simulink model "three_phase_bidirectional_EV_charger_simscape"  (R2019a)
settings: Solver=ode23tb  StartTime=0.0  StopTime=0.2  MaxStep=1e-5  RelTol=1e-5
values from neighbouring files (symbols this model uses):
  C = 33e-6    (= 3.3e-05)    [parameters_for_g2v_closed_loop.m]    (also in parameters_for_v2g_closed_loop.m = 0.002)
  Cf = 300e-3    (= 0.3)    [parameters_for_g2v_closed_loop.m]    (also in parameters_for_v2g_closed_loop.m)
  Co = 2e-3    (= 0.002)    [parameters_for_g2v_closed_loop.m]    (also in parameters_for_v2g_closed_loop.m)
  fline = 50    [parameters_for_g2v_closed_loop.m]    (also in parameters_for_v2g_closed_loop.m)
  fsw_dc = 100e3    (= 100000)    [parameters_for_g2v_closed_loop.m]    (also in parameters_for_v2g_closed_loop.m)
  H = 0.0075    [parameters_for_g2v_closed_loop.m]    (also in parameters_for_v2g_closed_loop.m)
  I = V/R    (= 10)    [parameters_for_g2v_closed_loop.m]    (also in parameters_for_v2g_closed_loop.m = V/(R*(1-D)))
  indicator = 1    [parameters_for_g2v_closed_loop.m]    (also in parameters_for_v2g_closed_loop.m = 0)
  Iqe_max = -Idc_max/K    (= -16.4102564103)    [parameters_for_g2v_closed_loop.m]    (also in parameters_for_v2g_closed_loop.m)
  Kic = Kpc/Tc    (= 4545.45454545)    [parameters_for_g2v_closed_loop.m]    (also in parameters_for_v2g_closed_loop.m)
  Kic_dc = 6749.8    [parameters_for_g2v_closed_loop.m]    (also in parameters_for_v2g_closed_loop.m = 9270.6)
  Kipll = Kpll/Tpll    [parameters_for_g2v_closed_loop.m]    (also in parameters_for_v2g_closed_loop.m)
  Kiv = Kpv/Tv_ac    [parameters_for_g2v_closed_loop.m]    (also in parameters_for_v2g_closed_loop.m)
  Kiv_dc = 15687    [parameters_for_g2v_closed_loop.m]    (also in parameters_for_v2g_closed_loop.m = 1260000)
  Kpc = Kc    (= 32.7272727273)    [parameters_for_g2v_closed_loop.m]    (also in parameters_for_v2g_closed_loop.m)
  Kpc_dc = 0.3    [parameters_for_g2v_closed_loop.m]    (also in parameters_for_v2g_closed_loop.m = 0.29)
  Kpll = (1/Vm)*(1/(alfa_pll*Tsamp_ac))    [parameters_for_g2v_closed_loop.m]    (also in parameters_for_v2g_closed_loop.m)
  Kpv = Kv    [parameters_for_g2v_closed_loop.m]    (also in parameters_for_v2g_closed_loop.m)
  Kpv_dc = 6.9    [parameters_for_g2v_closed_loop.m]    (also in parameters_for_v2g_closed_loop.m = 625.3)
  L = 250e-6    (= 0.00025)    [parameters_for_g2v_closed_loop.m]    (also in parameters_for_v2g_closed_loop.m)
  Lg = 1e-3    (= 0.001)    [parameters_for_g2v_closed_loop.m]    (also in parameters_for_v2g_closed_loop.m)
  Li = 1.6e-3    (= 0.0016)    [parameters_for_g2v_closed_loop.m]    (also in parameters_for_v2g_closed_loop.m)
  Ls = 1e-3    (= 0.001)    [parameters_for_g2v_closed_loop.m]    (also in parameters_for_v2g_closed_loop.m)
  R = V/Iload    (= 50)    [parameters_for_g2v_closed_loop.m]    (also in parameters_for_v2g_closed_loop.m = 1000000)
  Resr = 6e-3    (= 0.006)    [parameters_for_g2v_closed_loop.m]    (also in parameters_for_v2g_closed_loop.m = 0)
  Rf = 0.25    [parameters_for_g2v_closed_loop.m]    (also in parameters_for_v2g_closed_loop.m)
  RL = 10e-3    (= 0.01)    [parameters_for_g2v_closed_loop.m]    (also in parameters_for_v2g_closed_loop.m)
  Rs = 0.5    [parameters_for_g2v_closed_loop.m]    (also in parameters_for_v2g_closed_loop.m)
  T1 = Tsamp_ac/10    (= 5e-06)    [parameters_for_g2v_closed_loop.m]    (also in parameters_for_v2g_closed_loop.m)
  T2 = Tsamp_ac/10    (= 5e-06)    [parameters_for_g2v_closed_loop.m]    (also in parameters_for_v2g_closed_loop.m)
  Tsamp_ac = Tsw_ac/2    (= 5e-05)    [parameters_for_g2v_closed_loop.m]    (also in parameters_for_v2g_closed_loop.m)
  Tsamp_dc = Tsw_dc/2    (= 5e-06)    [parameters_for_g2v_closed_loop.m]    (also in parameters_for_v2g_closed_loop.m)
  V = 500    [parameters_for_g2v_closed_loop.m]    (also in parameters_for_v2g_closed_loop.m = 800)
  Vdc = 800    [parameters_for_g2v_closed_loop.m]    (also in parameters_for_v2g_closed_loop.m)
  Vm = 325    [parameters_for_g2v_closed_loop.m]    (also in parameters_for_v2g_closed_loop.m)
  VM = 4    [parameters_for_g2v_closed_loop.m]    (also in parameters_for_v2g_closed_loop.m)
undefined symbols (not defined in the file or in its folder): Ion, Lithium
libraries: powerlib x58, simulink x9, powerlib_meascontrol x1, electricdrivelib x1
(part 2 of 2)

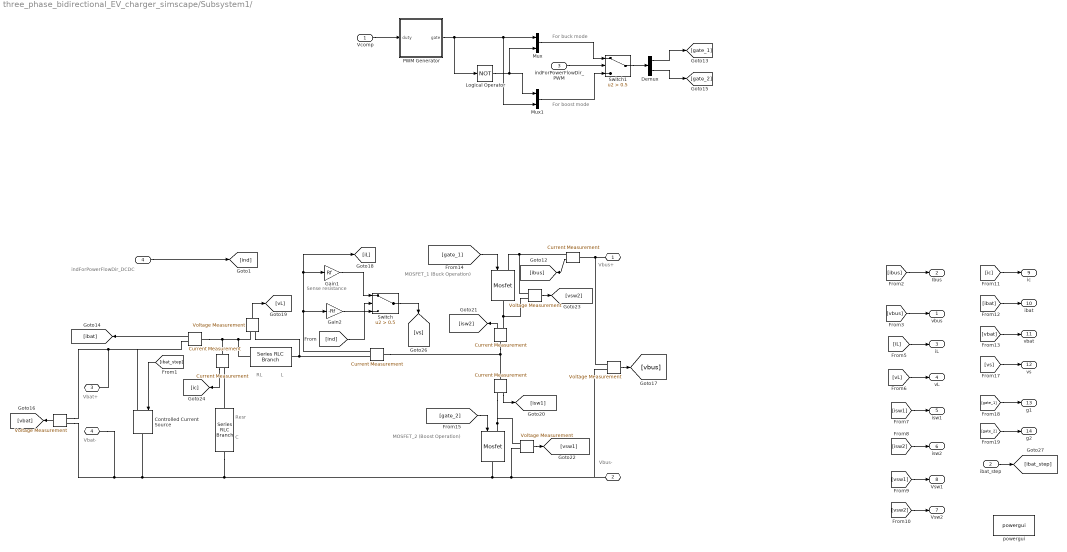
== system three_phase_bidirectional_EV_charger_simscape/Subsystem1/    ==
  note: For buck mode
  note: MOSFET_1
      | (Buck Operation)
  note: MOSFET_2
      | (Boost Operation)
  note: C
  note: Resr
  note: RL
  note: L
  note: Vbat+
  note: Vbat-
  note: Vbus+
  note: Vbus-
  note: For boost mode
  note: indForPowerFlowDir_DCDC
  note: Sense
      | resistance
  Vcomp : Inport
  ibat_step : Inport  Port=2
  indForPowerFlowDir_PWM : Inport  Port=3
  " " : Inport  Port=4
  " " : powerlib/Power Electronics/Mosfet  Ron=Rdson  Lon=0  Rd=0  Vfd=Vf  IC=0  Rs=1e5  Cs=inf  Measurements=off
      settings: SourceProductName=Simscape Electrical
   {,,,} (4 alike) : powerlib/Measurements/Voltage Measurement  PhasorSimulation=off  OutputType=Complex  PSBequivalent=0
      settings: SourceProductName=Simscape Electrical
   {,,,} (4 alike) : powerlib/Measurements/Current Measurement  PhasorSimulation=off  OutputType=Complex  PSBequivalent=0
      settings: SourceProductName=Simscape Electrical
  "    " : powerlib/Elements/Series RLC Branch  LConnTagsString=__new0  RConnTagsString=__new0  BranchType=RC  Resistance=Resr  Inductance=1e-3  SetiL0=off  InitialCurrent=0  Capacitance=C  Setx0=off  InitialVoltage=0  Measurements=None
      settings: SourceProductName=Simscape Electrical
  "        " : powerlib/Measurements/Current Measurement  PhasorSimulation=off  OutputType=Complex  PSBequivalent=0
      settings: SourceProductName=Simscape Electrical
  "          " : powerlib/Power Electronics/Mosfet  Ron=Rdson  Lon=0  Rd=0  Vfd=Vf  IC=0  Rs=1e5  Cs=inf  Measurements=off
      settings: SourceProductName=Simscape Electrical
  " " : powerlib/Elements/Series RLC Branch  LConnTagsString=__new0  RConnTagsString=__new0  BranchType=RL  Resistance=RL  Inductance=L  SetiL0=off  InitialCurrent=0  Capacitance=1e-6  Setx0=off  InitialVoltage=0  Measurements=None
      settings: SourceProductName=Simscape Electrical
  "                                                                                 " : powerlib/Measurements/Current Measurement  PhasorSimulation=off  OutputType=Complex  PSBequivalent=0
      settings: SourceProductName=Simscape Electrical
  "                                                                                                                                        " : powerlib/Measurements/Voltage Measurement  PhasorSimulation=off  OutputType=Complex  PSBequivalent=0
      settings: SourceProductName=Simscape Electrical
  Controlled Current Source : powerlib/Electrical Sources/Controlled Current Source  Initialize=off  Source_Type=AC  Amplitude=0  Phase=0  Frequency=0  Measurements=None
      settings: SourceProductName=Simscape Electrical
  Demux : Demux  Outputs=2
  Gain1 : Gain  Gain=Rf
  Gain2 : Gain  Gain=-Rf
  Logical Operator : Logic  Operator=NOT  AllPortsSameDT=off  OutDataTypeStr=boolean
  Mux : Mux  Inputs=2
  Mux1 : Mux  Inputs=2
  PWM Generator : Subsystem
  Switch : Switch  Criteria=u2 > Threshold  Threshold=0.5
  Switch1 : Switch  Criteria=u2 > Threshold  Threshold=0.5
  powergui : powerlib/powergui  Priority=1  SimulationMode=Continuous  SampleTime=50e-6  frequency=60  Iterations=50  frequencyindice=0  Pbase=100e6  ErrMax=1e-4  UnitsV=kV  UnitsW=MW  buscounter=0  FunctionMessages=off  echomessages=off  EnableUseOfTLC=off  CurrentSourceSwitches=off  DisableSnubberDevices=off  DisableRonSwitches=off  DisableVfSwitches=off  DisplayEquations=off  AutomaticDiscreteSolvers=off  SolverType=Tustin/Backward Euler (TBE)  Interpol=off  ExternalGateDelay=off  methode=off  Ts=100  x0status=blocks  SPID=on  SwTol=0  HookPort=off  NonlinearTolerance=0  nMaxIteration=15  ContinueOnMaxIteration=off  RestoreLinks=warning  ResistiveCurrentMeasurement=off  Frange=[0:2:500]  Ylog=off  Xlog=on  ShowGrid=off  save=off  variable=ZData  structure=0  ZoomFFT=off  StartTime=0.0  cycles=1  DisplayStyle=1  fundamental=60  FreqAxis=off  MaxFrequency=1000  frequencyindicesteady=1  RmsSteady=1  display=off
      settings: SourceProductName=Simscape Electrical
  "                                                                      " : PMIOPort  Side=Left
  "                                                                                                         " : PMIOPort  Port=2  Side=Left
  "                                                " : PMIOPort  Port=3  Side=Left
  "                                                                                                       " : PMIOPort  Port=4  Side=Left
  vbus : Outport
  Ibus : Outport  Port=2
  iL : Outport  Port=3
  vL : Outport  Port=4
  isw1 : Outport  Port=5
  isw2 : Outport  Port=6
  Vsw2 : Outport  Port=7
  Vsw1 : Outport  Port=8
  ic : Outport  Port=9
  ibat : Outport  Port=10
  vbat : Outport  Port=11
  vs : Outport  Port=12
  g1 : Outport  Port=13
  g2 : Outport  Port=14
  wires:
  Vcomp/1 -> PWM Generator/1(duty)
  [ibus] -> Ibus/1
  [vbus] -> vbus/1
  [iL] -> iL/1
  [vL] -> vL/1
  [isw1] -> isw1/1
  [isw2] -> isw2/1
  [vsw1] -> Vsw1/1
  [vsw2] -> Vsw2/1
  [ic] -> ic/1
  [ibat] -> ibat/1
  [vbat] -> vbat/1
  [gate_1] -> " "/1
  " "/1 -> [vsw2]
  [gate_2] -> "          "/1
  " "/1 -> [vL]
  " "/1 -> [vsw1]
  " "/1 -> [isw1]
  " "/1 -> [isw2]
  " "/1 -> [vbus]
  "                                                                                                                                        "/1 -> [vbat]
  " "/1 -> [ic]
  [vs] -> vs/1
  [gate_2] -> g2/1
  [gate_1] -> g1/1
  ibat_step/1 -> [ibat_step]
  "        "/1 -> [ibat]
  "                                                                                 "/1 -> [ibus]
  " "/1 -> Gain2/1, [iL], Gain1/1
  Gain1/1 -> Switch/1
  Switch/1 -> [vs]
  Gain2/1 -> Switch/3
  PWM Generator/1(gate) -> Mux/1, Mux1/2, Logical Operator/1
  Logical Operator/1 -> Mux1/1, Mux/2
  Mux/1 -> Switch1/1
  Mux1/1 -> Switch1/3
  Switch1/1 -> Demux/1
  Demux/1 -> [gate_1]
  Demux/2 -> [gate_2]
  indForPowerFlowDir_PWM/1 -> Switch1/2
  " "/1 -> [ind]
  [ind] -> Switch/2
  [ibat_step] -> Controlled Current Source/1
  connections:
  " "/RConn1 -- " "/LConn1
  "          "/LConn1 -- " "/RConn1 -- " "/LConn1
  " "/LConn1 -- ?
  " "/LConn2 -- " "/RConn1
  "                                                                                                                                        "/LConn1 -- Controlled Current Source/LConn1 -- "        "/RConn1 -- "                                                "/RConn1
  " "/LConn1 -- "                                                                                 "/LConn1 -- "                                                                      "/RConn1
  "                                                                                                                                        "/LConn2 -- "                                                                                                       "/RConn1 -- Controlled Current Source/RConn1 -- "                                                                                                         "/RConn1 -- " "/LConn2 -- "          "/RConn1 -- "    "/RConn1
  " "/LConn1 -- "        "/LConn1
  " "/LConn2 -- "                                                                                 "/RConn1 -- " "/LConn1
  "    "/LConn1 -- " "/RConn1

== system three_phase_bidirectional_EV_charger_simscape/Subsystem1/Battery load step g2v ==
  Add : Sum
  Step : Step  Time=0.045  After=-V/(1.5*R)  SampleTime=0
  Step1 : Step  Time=0.06  After=V/(1.5*R)  SampleTime=0
  Iload_step : Outport
  wires:
  Add/1 -> Iload_step/1
  Step/1 -> Add/1
  Step1/1 -> Add/2

== system three_phase_bidirectional_EV_charger_simscape/Subsystem1/Battery load step v2g ==
  step : Constant  Value=0
  Iload_step : Outport
  wires:
  step/1 -> Iload_step/1

== system three_phase_bidirectional_EV_charger_simscape/Subsystem1/Controller - Boost Mode ==
  Vs : Inport
  Vo_meas : Inport  Port=2
  Vref : Inport  Port=3
  Current Compensator : Subsystem
  "Voltage Compensator " : Subsystem
  "Vcomp " : Outport
  wires:
  Vs/1 -> Current Compensator/1(Vs)
  "Voltage Compensator "/1(Vc) -> Current Compensator/2(Vc)
  Vref/1 -> "Voltage Compensator "/2(Vref)
  Current Compensator/1(Vcomp) -> "Vcomp "/1
  Vo_meas/1 -> "Voltage Compensator "/1("Vo_meas ")

== system three_phase_bidirectional_EV_charger_simscape/Subsystem1/Controller - Buck Mode ==
  Vs : Inport
  Vo_meas : Inport  Port=2
  Vref : Inport  Port=3
  Current PI Compensator : Subsystem
  "Voltage PI Compensator " : Subsystem
  "Vcomp " : Outport
  wires:
  Vs/1 -> Current PI Compensator/1(Vs)
  "Voltage PI Compensator "/1(Vc) -> Current PI Compensator/2(Vc)
  Vref/1 -> "Voltage PI Compensator "/2(Vref)
  Current PI Compensator/1(Vcomp) -> "Vcomp "/1
  Vo_meas/1 -> "Voltage PI Compensator "/1("Vo_meas ")

== system three_phase_bidirectional_EV_charger_simscape/Subsystem1/DC link variation v2g ==
  Add : Sum
  Step : Step  Time=0.015  After=-H*1.2  SampleTime=0
  Step1 : Step  Time=0.03  After=H*1.2  SampleTime=0
  Vbus_step : Outport
  wires:
  Step1/1 -> Add/2
  Step/1 -> Add/1
  Add/1 -> Vbus_step/1

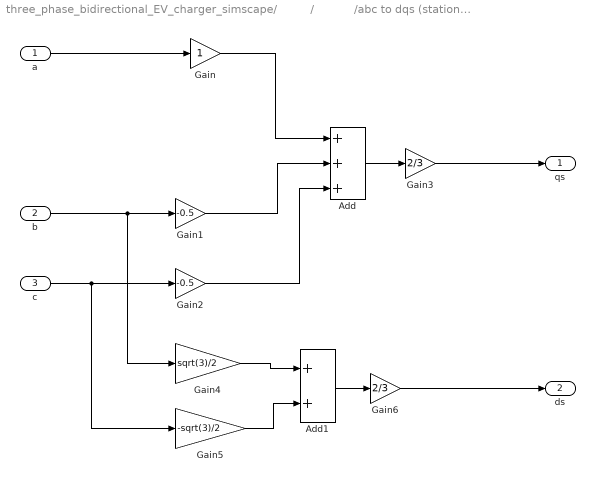
== system three_phase_bidirectional_EV_charger_simscape/          /            /abc to dqs (stationary) ==
  a : Inport
  b : Inport  Port=2
  c : Inport  Port=3
  Add : Sum  Inputs=+++
  Add1 : Sum
  Gain : Gain
  Gain1 : Gain  Gain=-0.5
  Gain2 : Gain  Gain=-0.5
  Gain3 : Gain  Gain=2/3
  Gain4 : Gain  Gain=sqrt(3)/2
  Gain5 : Gain  Gain=-sqrt(3)/2
  Gain6 : Gain  Gain=2/3
  qs : Outport
  ds : Outport  Port=2
  wires:
  a/1 -> Gain/1
  Gain/1 -> Add/1
  Gain5/1 -> Add1/2
  Gain1/1 -> Add/2
  b/1 -> Gain4/1, Gain1/1
  c/1 -> Gain5/1, Gain2/1
  Add/1 -> Gain3/1
  Gain2/1 -> Add/3
  Gain4/1 -> Add1/1
  Gain3/1 -> qs/1
  Add1/1 -> Gain6/1
  Gain6/1 -> ds/1

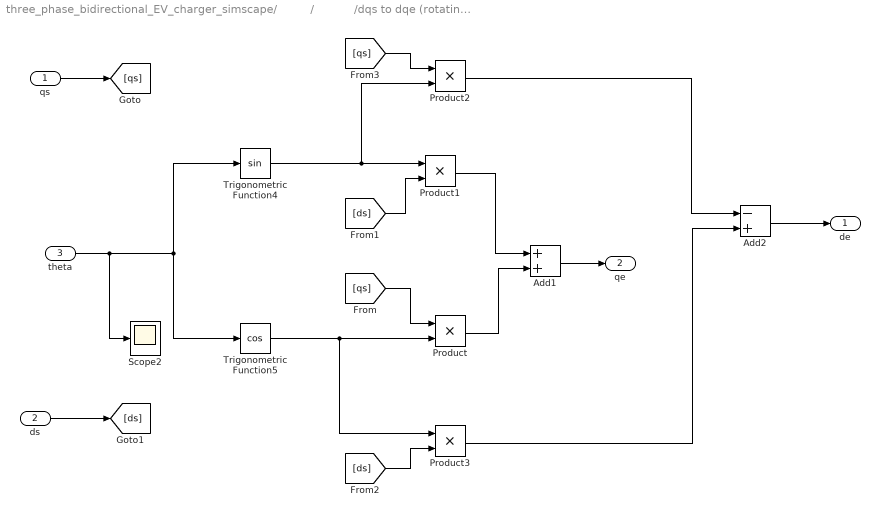
== system three_phase_bidirectional_EV_charger_simscape/          /            /dqs to dqe (rotating) ==
  "qs " : Inport
  "ds " : Inport  Port=2
  theta : Inport  Port=3
  Add1 : Sum
  Add2 : Sum  Inputs=-+
  Product{,1..3} (4 alike) : Product
  Scope2 : Scope
  Trigonometric Function4 : Trigonometry
  Trigonometric Function5 : Trigonometry  Operator=cos
  "de " : Outport
  "qe " : Outport  Port=2
  wires:
  [ds] -> Product3/2
  theta/1 -> Scope2/1, Trigonometric Function4/1, Trigonometric Function5/1
  "ds "/1 -> [ds]
  Add2/1 -> "de "/1
  Product2/1 -> Add2/1
  [qs] -> Product/1
  "qs "/1 -> [qs]
  Product3/1 -> Add2/2
  [qs] -> Product2/1
  Add1/1 -> "qe "/1
  [ds] -> Product1/2
  Product/1 -> Add1/2
  Product1/1 -> Add1/1
  Trigonometric Function4/1 -> Product2/2, Product1/1
  Trigonometric Function5/1 -> Product/2, Product3/1

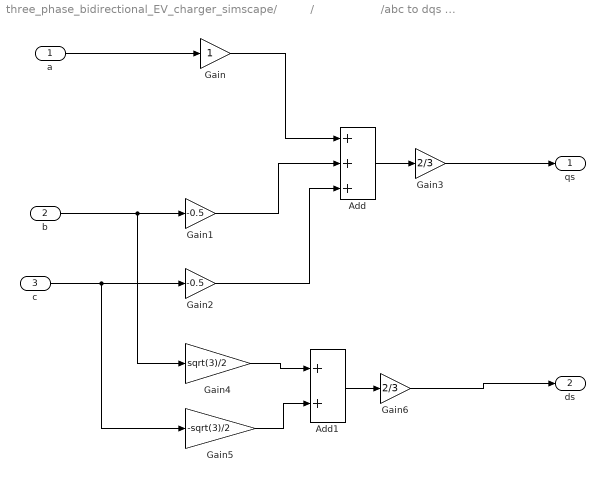
== system three_phase_bidirectional_EV_charger_simscape/          /                    /abc to dqs (stationary) ==
  a : Inport
  b : Inport  Port=2
  c : Inport  Port=3
  Add : Sum  Inputs=+++
  Add1 : Sum
  Gain : Gain
  Gain1 : Gain  Gain=-0.5
  Gain2 : Gain  Gain=-0.5
  Gain3 : Gain  Gain=2/3
  Gain4 : Gain  Gain=sqrt(3)/2
  Gain5 : Gain  Gain=-sqrt(3)/2
  Gain6 : Gain  Gain=2/3
  qs : Outport
  ds : Outport  Port=2
  wires:
  a/1 -> Gain/1
  Gain/1 -> Add/1
  Gain5/1 -> Add1/2
  Gain1/1 -> Add/2
  b/1 -> Gain4/1, Gain1/1
  c/1 -> Gain5/1, Gain2/1
  Add/1 -> Gain3/1
  Gain2/1 -> Add/3
  Gain4/1 -> Add1/1
  Gain3/1 -> qs/1
  Add1/1 -> Gain6/1
  Gain6/1 -> ds/1

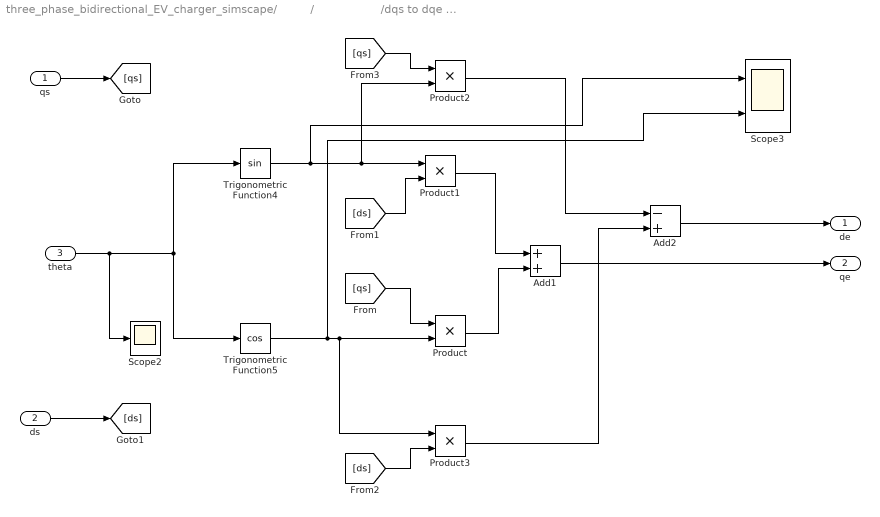
== system three_phase_bidirectional_EV_charger_simscape/          /                    /dqs to dqe (rotating) ==
  "qs " : Inport
  "ds " : Inport  Port=2
  theta : Inport  Port=3
  Add1 : Sum
  Add2 : Sum  Inputs=-+
  Product{,1..3} (4 alike) : Product
  Scope2 : Scope
  Scope3 : Scope  NumInputPorts=2
  Trigonometric Function4 : Trigonometry
  Trigonometric Function5 : Trigonometry  Operator=cos
  "de " : Outport
  "qe " : Outport  Port=2
  wires:
  [ds] -> Product3/2
  theta/1 -> Scope2/1, Trigonometric Function4/1, Trigonometric Function5/1
  "ds "/1 -> [ds]
  Add2/1 -> "de "/1
  Product2/1 -> Add2/1
  [qs] -> Product/1
  "qs "/1 -> [qs]
  Product3/1 -> Add2/2
  [qs] -> Product2/1
  Add1/1 -> "qe "/1
  [ds] -> Product1/2
  Product/1 -> Add1/2
  Product1/1 -> Add1/1
  Trigonometric Function4/1 -> Product2/2, Product1/1, Scope3/1
  Trigonometric Function5/1 -> Product/2, Product3/1, Scope3/2

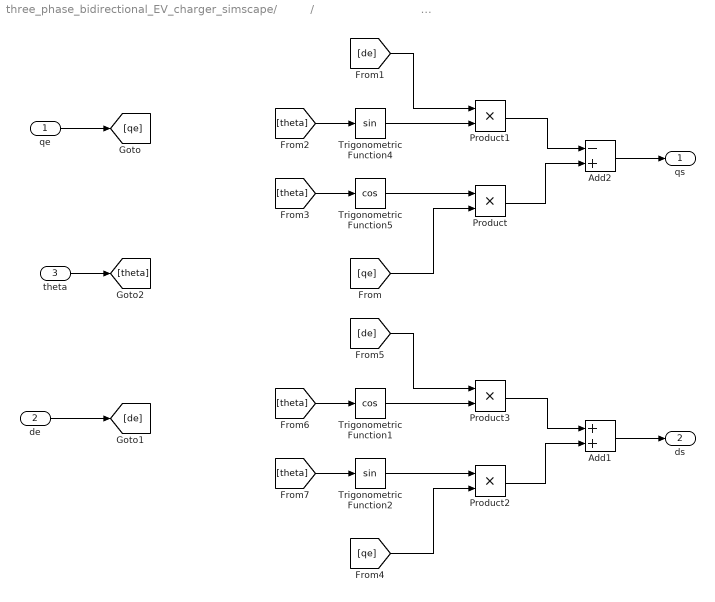
== system three_phase_bidirectional_EV_charger_simscape/          /                                                                                                                                                                                                                                                   /dqe to dqs ==
  "qe " : Inport
  "de " : Inport  Port=2
  theta : Inport  Port=3
  Add1 : Sum
  Add2 : Sum  Inputs=-+
  Product{,1..3} (4 alike) : Product
  Trigonometric Function1 : Trigonometry  Operator=cos
  Trigonometric Function2 : Trigonometry
  Trigonometric Function4 : Trigonometry
  Trigonometric Function5 : Trigonometry  Operator=cos
  "qs " : Outport
  ds : Outport  Port=2
  wires:
  "de "/1 -> [de]
  Add2/1 -> "qs "/1
  "qe "/1 -> [qe]
  Trigonometric Function5/1 -> Product/1
  [qe] -> Product/2
  Trigonometric Function4/1 -> Product1/2
  [de] -> Product1/1
  Product1/1 -> Add2/1
  Product/1 -> Add2/2
  theta/1 -> [theta]
  [theta] -> Trigonometric Function4/1
  [theta] -> Trigonometric Function5/1
  Trigonometric Function1/1 -> Product3/2
  [theta] -> Trigonometric Function2/1
  [theta] -> Trigonometric Function1/1
  Product2/1 -> Add1/2
  [de] -> Product3/1
  [qe] -> Product2/2
  Trigonometric Function2/1 -> Product2/1
  Add1/1 -> ds/1
  Product3/1 -> Add1/1

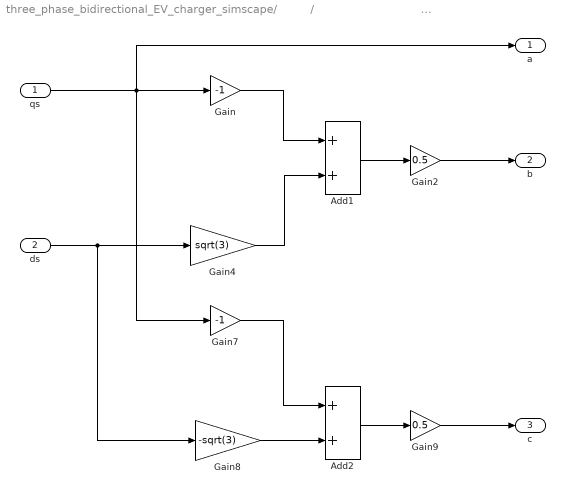
== system three_phase_bidirectional_EV_charger_simscape/          /                                                                                                                                                                                                                                                   /dqs to abc ==
  qs : Inport
  ds : Inport  Port=2
  Add1 : Sum
  Add2 : Sum
  Gain : Gain  Gain=-1
  Gain2 : Gain  Gain=0.5
  Gain4 : Gain  Gain=sqrt(3)
  Gain7 : Gain  Gain=-1
  Gain8 : Gain  Gain=-sqrt(3)
  Gain9 : Gain  Gain=0.5
  a : Outport
  b : Outport  Port=2
  c : Outport  Port=3
  wires:
  qs/1 -> Gain7/1, a/1, Gain/1
  ds/1 -> Gain8/1, Gain4/1
  Gain/1 -> Add1/1
  Gain4/1 -> Add1/2
  Add1/1 -> Gain2/1
  Gain2/1 -> b/1
  Gain7/1 -> Add2/1
  Gain8/1 -> Add2/2
  Add2/1 -> Gain9/1
  Gain9/1 -> c/1

== system three_phase_bidirectional_EV_charger_simscape/Subsystem1/   /PWM Generator ==
  duty : Inport
  Relational Operator : RelationalOperator  Operator=<=  OutDataTypeStr=boolean  RndMeth=Simplest
  Repeating Sequence : simulink/Sources/Repeating Sequence  rep_seq_t=[0 0.5/fsw_dc 1/fsw_dc]  rep_seq_y=[0 VM 0]
  gate : Outport
  wires:
  Repeating Sequence/1 -> Relational Operator/1
  Relational Operator/1 -> gate/1
  duty/1 -> Relational Operator/2

== system three_phase_bidirectional_EV_charger_simscape/Subsystem1/Controller - Boost Mode/Current Compensator ==
  Vs : Inport
  Vc : Inport  Port=2
  PID Controller : simulink/Continuous/PID Controller  Controller=PI  Form=Parallel  TimeDomain=Continuous-time  SampleTime=-1  IntegratorMethod=Forward Euler  FilterMethod=Forward Euler  ControllerParametersSource=internal  P=Kpc_dc  I=Kic_dc  D=0  UseFilter=on  N=100  TunerSelectOption=Transfer Function Based (PID Tuner App)  InitialConditionSource=internal  InitialConditionForIntegrator=0  InitialConditionForFilter=0  DifferentiatorICPrevScaledInput=0  ExternalReset=none  TrackingMode=off  Kt=1  LimitOutput=off  UpperSaturationLimit=VM  LowerSaturationLimit=-VM  LinearizeAsGain=on  AntiWindupMode=none  Kb=1  POutMin=[]  POutMax=[]  IOutMin=[]  IOutMax=[]  DOutMin=[]  DOutMax=[]  NOutMin=[]  NOutMax=[]  SumOutMin=[]  SumOutMax=[]  SaturationOutMin=[]  SaturationOutMax=[]  PParamMin=[]  PParamMax=[]  IParamMin=[]  IParamMax=[]  DParamMin=[]  DParamMax=[]  NParamMin=[]  NParamMax=[]  KbParamMin=[]  KbParamMax=[]  KtParamMin=[]  KtParamMax=[]  KbOutMin=[]  KbOutMax=[]  KtOutMin=[]  KtOutMax=[]  IntegratorOutMin=[]  IntegratorOutMax=[]  FilterOutMin=[]  FilterOutMax=[]  SumI1OutMin=[]  SumI1OutMax=[]  SumI2OutMin=[]  SumI2OutMax=[]  SumI3OutMin=[]  SumI3OutMax=[]  SumI4OutMin=[]  SumI4OutMax=[]  SumDOutMin=[]  SumDOutMax=[]  DifferentiatorOutMin=[]  DifferentiatorOutMax=[]  FilterDiffOutCoefMin=[]  FilterDiffOutCoefMax=[]  ReciprocalOutMin=[]  ReciprocalOutMax=[]  SumDenOutMin=[]  SumDenOutMax=[]  SumNumOutMin=[]  SumNumOutMax=[]  DivideOutMin=[]  DivideOutMax=[]  IntegratorContinuousStateAttributes=''  IntegratorStateMustResolveToSignalObject=off  IntegratorRTWStateStorageClass=Auto  FilterContinuousStateAttributes=''  FilterStateMustResolveToSignalObject=off  FilterRTWStateStorageClass=Auto  ParallelPVariant=InternalParameters  IdealPVariant=Disabled  IVariant=InternalParameters  DVariant=Disabled  IntegratorVariant=Continuous  SatVariant=Disabled  AWVariant=Passthrough  PCopyVariant=Disabled  TRVariant=Disabled  FdbkBlocksVariant=Forward  IdealPFdbkVariant=Disabled  SatFdbkVariant=Disabled  DerivativeFilterVariant=Disabled  NVariant=Disabled  NCopyVariant=Disabled_SignalSpec  FilterICVariant=Disabled  IntegratorICVariant=InternalICs  ExternalResetVariant=Disabled  TRSumVariant=Passthrough  SumFdbkVariant=Disabled  SumVariant=Sum_PI
  Sum : Sum  Inputs=|+-
  Transfer Fcn6 : TransferFcn  Denominator=[Tsamp_dc 1]
  Vcomp : Outport
  wires:
  Vc/1 -> Sum/1
  Vs/1 -> Sum/2
  Sum/1 -> Transfer Fcn6/1
  Transfer Fcn6/1 -> PID Controller/1
  PID Controller/1 -> Vcomp/1

== system three_phase_bidirectional_EV_charger_simscape/Subsystem1/Controller - Boost Mode/Voltage Compensator  ==
  "Vo_meas " : Inport
  Vref : Inport  Port=2
  PID Controller : simulink/Continuous/PID Controller  Controller=PI  Form=Parallel  TimeDomain=Continuous-time  SampleTime=-1  IntegratorMethod=Forward Euler  FilterMethod=Forward Euler  ControllerParametersSource=internal  P=Kpv_dc  I=Kiv_dc  D=0  UseFilter=on  N=100  TunerSelectOption=Transfer Function Based (PID Tuner App)  InitialConditionSource=internal  InitialConditionForIntegrator=0  InitialConditionForFilter=0  DifferentiatorICPrevScaledInput=0  ExternalReset=none  TrackingMode=off  Kt=1  LimitOutput=off  UpperSaturationLimit=2.5*Rf*I  LowerSaturationLimit=-2.5*Rf*I  LinearizeAsGain=on  AntiWindupMode=none  Kb=1  POutMin=[]  POutMax=[]  IOutMin=[]  IOutMax=[]  DOutMin=[]  DOutMax=[]  NOutMin=[]  NOutMax=[]  SumOutMin=[]  SumOutMax=[]  SaturationOutMin=[]  SaturationOutMax=[]  PParamMin=[]  PParamMax=[]  IParamMin=[]  IParamMax=[]  DParamMin=[]  DParamMax=[]  NParamMin=[]  NParamMax=[]  KbParamMin=[]  KbParamMax=[]  KtParamMin=[]  KtParamMax=[]  KbOutMin=[]  KbOutMax=[]  KtOutMin=[]  KtOutMax=[]  IntegratorOutMin=[]  IntegratorOutMax=[]  FilterOutMin=[]  FilterOutMax=[]  SumI1OutMin=[]  SumI1OutMax=[]  SumI2OutMin=[]  SumI2OutMax=[]  SumI3OutMin=[]  SumI3OutMax=[]  SumI4OutMin=[]  SumI4OutMax=[]  SumDOutMin=[]  SumDOutMax=[]  DifferentiatorOutMin=[]  DifferentiatorOutMax=[]  FilterDiffOutCoefMin=[]  FilterDiffOutCoefMax=[]  ReciprocalOutMin=[]  ReciprocalOutMax=[]  SumDenOutMin=[]  SumDenOutMax=[]  SumNumOutMin=[]  SumNumOutMax=[]  DivideOutMin=[]  DivideOutMax=[]  IntegratorContinuousStateAttributes=''  IntegratorStateMustResolveToSignalObject=off  IntegratorRTWStateStorageClass=Auto  FilterContinuousStateAttributes=''  FilterStateMustResolveToSignalObject=off  FilterRTWStateStorageClass=Auto  ParallelPVariant=InternalParameters  IdealPVariant=Disabled  IVariant=InternalParameters  DVariant=Disabled  IntegratorVariant=Continuous  SatVariant=Disabled  AWVariant=Passthrough  PCopyVariant=Disabled  TRVariant=Disabled  FdbkBlocksVariant=Forward  IdealPFdbkVariant=Disabled  SatFdbkVariant=Disabled  DerivativeFilterVariant=Disabled  NVariant=Disabled  NCopyVariant=Disabled_SignalSpec  FilterICVariant=Disabled  IntegratorICVariant=InternalICs  ExternalResetVariant=Disabled  TRSumVariant=Passthrough  SumFdbkVariant=Disabled  SumVariant=Sum_PI
  Sum : Sum  Inputs=|+-
  Vc : Outport
  wires:
  "Vo_meas "/1 -> Sum/2
  Vref/1 -> Sum/1
  Sum/1 -> PID Controller/1
  PID Controller/1 -> Vc/1

== system three_phase_bidirectional_EV_charger_simscape/Subsystem1/Controller - Buck Mode/Current PI Compensator ==
  Vs : Inport
  Vc : Inport  Port=2
  PID Controller : simulink/Continuous/PID Controller  Controller=PI  Form=Parallel  TimeDomain=Continuous-time  SampleTime=-1  IntegratorMethod=Forward Euler  FilterMethod=Forward Euler  ControllerParametersSource=internal  P=Kpc_dc  I=Kic_dc  D=0  UseFilter=on  N=100  TunerSelectOption=Transfer Function Based (PID Tuner App)  InitialConditionSource=internal  InitialConditionForIntegrator=0  InitialConditionForFilter=0  DifferentiatorICPrevScaledInput=0  ExternalReset=none  TrackingMode=off  Kt=1  LimitOutput=off  UpperSaturationLimit=VM  LowerSaturationLimit=0  LinearizeAsGain=on  AntiWindupMode=none  Kb=1  POutMin=[]  POutMax=[]  IOutMin=[]  IOutMax=[]  DOutMin=[]  DOutMax=[]  NOutMin=[]  NOutMax=[]  SumOutMin=[]  SumOutMax=[]  SaturationOutMin=[]  SaturationOutMax=[]  PParamMin=[]  PParamMax=[]  IParamMin=[]  IParamMax=[]  DParamMin=[]  DParamMax=[]  NParamMin=[]  NParamMax=[]  KbParamMin=[]  KbParamMax=[]  KtParamMin=[]  KtParamMax=[]  KbOutMin=[]  KbOutMax=[]  KtOutMin=[]  KtOutMax=[]  IntegratorOutMin=[]  IntegratorOutMax=[]  FilterOutMin=[]  FilterOutMax=[]  SumI1OutMin=[]  SumI1OutMax=[]  SumI2OutMin=[]  SumI2OutMax=[]  SumI3OutMin=[]  SumI3OutMax=[]  SumI4OutMin=[]  SumI4OutMax=[]  SumDOutMin=[]  SumDOutMax=[]  DifferentiatorOutMin=[]  DifferentiatorOutMax=[]  FilterDiffOutCoefMin=[]  FilterDiffOutCoefMax=[]  ReciprocalOutMin=[]  ReciprocalOutMax=[]  SumDenOutMin=[]  SumDenOutMax=[]  SumNumOutMin=[]  SumNumOutMax=[]  DivideOutMin=[]  DivideOutMax=[]  IntegratorContinuousStateAttributes=''  IntegratorStateMustResolveToSignalObject=off  IntegratorRTWStateStorageClass=Auto  FilterContinuousStateAttributes=''  FilterStateMustResolveToSignalObject=off  FilterRTWStateStorageClass=Auto  ParallelPVariant=InternalParameters  IdealPVariant=Disabled  IVariant=InternalParameters  DVariant=Disabled  IntegratorVariant=Continuous  SatVariant=Disabled  AWVariant=Passthrough  PCopyVariant=Disabled  TRVariant=Disabled  FdbkBlocksVariant=Forward  IdealPFdbkVariant=Disabled  SatFdbkVariant=Disabled  DerivativeFilterVariant=Disabled  NVariant=Disabled  NCopyVariant=Disabled_SignalSpec  FilterICVariant=Disabled  IntegratorICVariant=InternalICs  ExternalResetVariant=Disabled  TRSumVariant=Passthrough  SumFdbkVariant=Disabled  SumVariant=Sum_PI
  Sum : Sum  Inputs=|+-
  Transfer Fcn6 : TransferFcn  Denominator=[Tsamp_dc 1]
  Vcomp : Outport
  wires:
  Vc/1 -> Sum/1
  Vs/1 -> Sum/2
  Sum/1 -> Transfer Fcn6/1
  Transfer Fcn6/1 -> PID Controller/1
  PID Controller/1 -> Vcomp/1

== system three_phase_bidirectional_EV_charger_simscape/Subsystem1/Controller - Buck Mode/Voltage PI Compensator  ==
  "Vo_meas " : Inport
  Vref : Inport  Port=2
  PID Controller : simulink/Continuous/PID Controller  Controller=PI  Form=Parallel  TimeDomain=Continuous-time  SampleTime=-1  IntegratorMethod=Forward Euler  FilterMethod=Forward Euler  ControllerParametersSource=internal  P=Kpv_dc  I=Kiv_dc  D=0  UseFilter=on  N=100  TunerSelectOption=Transfer Function Based (PID Tuner App)  InitialConditionSource=internal  InitialConditionForIntegrator=0  InitialConditionForFilter=0  DifferentiatorICPrevScaledInput=0  ExternalReset=none  TrackingMode=off  Kt=1  LimitOutput=off  UpperSaturationLimit=40*Rf  LowerSaturationLimit=0  LinearizeAsGain=on  AntiWindupMode=none  Kb=1  POutMin=[]  POutMax=[]  IOutMin=[]  IOutMax=[]  DOutMin=[]  DOutMax=[]  NOutMin=[]  NOutMax=[]  SumOutMin=[]  SumOutMax=[]  SaturationOutMin=[]  SaturationOutMax=[]  PParamMin=[]  PParamMax=[]  IParamMin=[]  IParamMax=[]  DParamMin=[]  DParamMax=[]  NParamMin=[]  NParamMax=[]  KbParamMin=[]  KbParamMax=[]  KtParamMin=[]  KtParamMax=[]  KbOutMin=[]  KbOutMax=[]  KtOutMin=[]  KtOutMax=[]  IntegratorOutMin=[]  IntegratorOutMax=[]  FilterOutMin=[]  FilterOutMax=[]  SumI1OutMin=[]  SumI1OutMax=[]  SumI2OutMin=[]  SumI2OutMax=[]  SumI3OutMin=[]  SumI3OutMax=[]  SumI4OutMin=[]  SumI4OutMax=[]  SumDOutMin=[]  SumDOutMax=[]  DifferentiatorOutMin=[]  DifferentiatorOutMax=[]  FilterDiffOutCoefMin=[]  FilterDiffOutCoefMax=[]  ReciprocalOutMin=[]  ReciprocalOutMax=[]  SumDenOutMin=[]  SumDenOutMax=[]  SumNumOutMin=[]  SumNumOutMax=[]  DivideOutMin=[]  DivideOutMax=[]  IntegratorContinuousStateAttributes=''  IntegratorStateMustResolveToSignalObject=off  IntegratorRTWStateStorageClass=Auto  FilterContinuousStateAttributes=''  FilterStateMustResolveToSignalObject=off  FilterRTWStateStorageClass=Auto  ParallelPVariant=InternalParameters  IdealPVariant=Disabled  IVariant=InternalParameters  DVariant=Disabled  IntegratorVariant=Continuous  SatVariant=Disabled  AWVariant=Passthrough  PCopyVariant=Disabled  TRVariant=Disabled  FdbkBlocksVariant=Forward  IdealPFdbkVariant=Disabled  SatFdbkVariant=Disabled  DerivativeFilterVariant=Disabled  NVariant=Disabled  NCopyVariant=Disabled_SignalSpec  FilterICVariant=Disabled  IntegratorICVariant=InternalICs  ExternalResetVariant=Disabled  TRSumVariant=Passthrough  SumFdbkVariant=Disabled  SumVariant=Sum_PI
  Sum : Sum  Inputs=|+-
  Vc : Outport
  wires:
  "Vo_meas "/1 -> Sum/2
  Vref/1 -> Sum/1
  Sum/1 -> PID Controller/1
  PID Controller/1 -> Vc/1
